simulink model "LQR_SIP_v2"  (R2022b)
settings: Solver=ode4  StartTime=0.0  StopTime=60*5  FixedStep=0.002  RelTol=1e-3  EnableMultiTasking=on
PostLoadFcn:
  | qc_set_target_type(getConfigSet(bdroot, 'QUARC Default Target Configuration'));
undefined symbols (not defined in the file): ALPHA_MAX, ALPHA_MIN, HIL, K, K_EC, K_EP, qc_get_step_size, wcf, XC_MAX, XC_MIN, zetaf
libraries: quarc_library x9, simulink_extras x3
Description:
  | This example is a simple analog loopback test. It sends a signal to analog output
  | channel #0 and then reads analog input channel #0. Wire analog output #0 to analog
  | input #0 to see the signal on the Scope. Change the amplitude of the signal and see
  | the change occur on the Scope.
settings Model: SimulationMode=external  ExtModeTrigDuration=10000  Creator=drmadill  LastModifiedBy=tst2753
settings SolverCC: AlgebraicLoopSolver=TrustRegion  PositivePriorityOrder=on
settings DataIOCC: LimitDataPoints=on  SaveFormat=Array  SignalLoggingSaveFormat=ModelDataLogs  InspectSignalLogs=on  ReturnWorkspaceOutputs=off
settings OptimizationCC: ExpressionDepthLimit=2147483647  InitFltsAndDblsToZero=on
settings DebuggingCC: SaveWithParameterizedLinksMsg=none  UnderspecifiedInitializationDetection=Classic  MergeDetectMultiDrivingBlocksExec=none  SolverPrmCheckMsg=warning  FcnCallInpInsideContextMsg=warning  UnconnectedInputMsg=warning  UnconnectedOutputMsg=warning  UnconnectedLineMsg=warning  StateNameClashWarn=warning  SFUnexpectedBacktrackingDiag=warning  SFNoUnconditionalDefaultTransitionDiag=warning  SFMachineParentedDataDiag=warning  ArithmeticOperatorsInVariantConditions=warning
settings ModelReferenceCC: EnableRefExpFcnMdlSchedulingChecks=on  PropagateSignalLabelsOutOfModel=off
settings SFSimCC: SimUseLocalCustomCode=off  CustomCodeUndefinedFunction=UseInterfaceOnly
settings RTWCC: Description=QUARC Win64 Target Using Toolchain  SystemTargetFile=quarc_win64.tlc  TemplateMakefile=quarc_default_tmf  RTWUseLocalCustomCode=off  Toolchain=QUARC win64 | nmake (64-bit Windows)  BuildConfiguration=Faster Runs
settings CodeAppCC: StateflowObjectComments=on
settings STFCustomTargetCC: ConcurrentExecutionCompliant=on  GRTInterface=on  UseToolchainInfoCompliant=on  SystemTargetFile=quarc_win64.tlc
settings GRTTargetCC: TargetLangStandard=C89/C90 (ANSI)  ParMdlRefBuildCompliant=off  CompOptLevelCompliant=off  CombineOutputUpdateFcns=off  MatFileLogging=off  CPPClassGenCompliant=off  GRTInterface=on  ExtMode=on  ExtModeMexFile=quarc_comm
settings ConfigComp: CovMetricSettings=dw  CovSaveCumulativeToWorkspaceVar=on  CovSaveSingleToWorkspaceVar=on  CovExternalEMLEnable=off

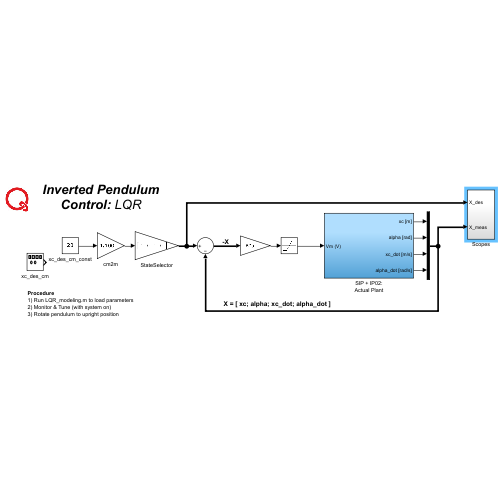
[thumbnail: Simulink's stored preview of the top-level diagram]
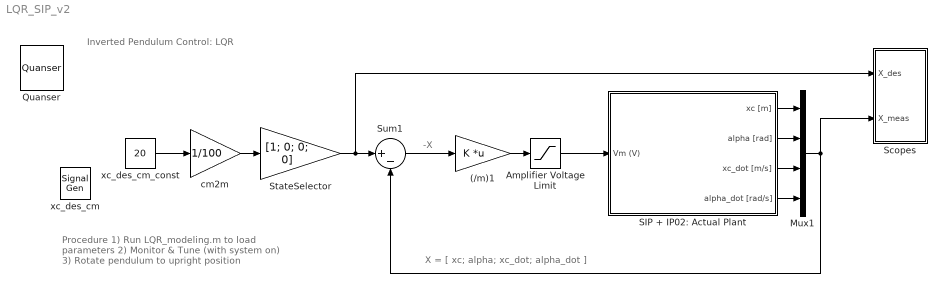
== system LQR_SIP_v2 ==
  note: X = [ xc; alpha; xc_dot; alpha_dot ]
  note: -X
  note: Procedure
      | 1) Run LQR_modeling.m to load parameters
      | 2) Monitor & Tune (with system on)
      | 3) Rotate pendulum to upright position
  note: Inverted Pendulum Control: LQR
  (/m)1 : Gain  Gain=K  Multiplication=Matrix(K*u)  SaturateOnIntegerOverflow=on  OutDataTypeStr=Inherit: Same as input  ParamDataTypeStr=Inherit: Same as input
  Amplifier Voltage Limit : Saturate  UpperLimit=10  LowerLimit=-10
  Mux1 : Mux
  Quanser : quarc_library/Logos/Quanser
  SIP + IP02: Actual Plant : Subsystem
  Scopes : Subsystem
  StateSelector : Gain  Gain=[1; 0; 0; 0]  SaturateOnIntegerOverflow=on  OutDataTypeStr=Inherit: Same as input  ParamDataTypeStr=Inherit: Same as input
  Sum1 : Sum  Inputs=|+-  InputSameDT=on  SaturateOnIntegerOverflow=on  OutDataTypeStr=Inherit: Same as first input
  cm2m : Gain  Gain=1/100  SaturateOnIntegerOverflow=on  OutDataTypeStr=Inherit: Same as input  ParamDataTypeStr=Inherit: Same as input
  xc_des_cm : SignalGenerator  Amplitude=20  Frequency=0.15
  xc_des_cm_const : Constant  Value=20
  wires:
  (/m)1/1 -> Amplifier Voltage Limit/1
  SIP + IP02: Actual Plant/3(xc_dot [m/s]) -> Mux1/3
  cm2m/1 -> StateSelector/1
  StateSelector/1 -> Sum1/1, Scopes/1(X_des)
  Amplifier Voltage Limit/1 -> SIP + IP02: Actual Plant/1(Vm (V))
  Sum1/1 -> (/m)1/1
  SIP + IP02: Actual Plant/4(alpha_dot [rad/s]) -> Mux1/4
  Mux1/1 -> Scopes/2(X_meas), Sum1/2
  SIP + IP02: Actual Plant/1(xc [m]) -> Mux1/1
  SIP + IP02: Actual Plant/2(alpha [rad]) -> Mux1/2
  xc_des_cm_const/1 -> cm2m/1

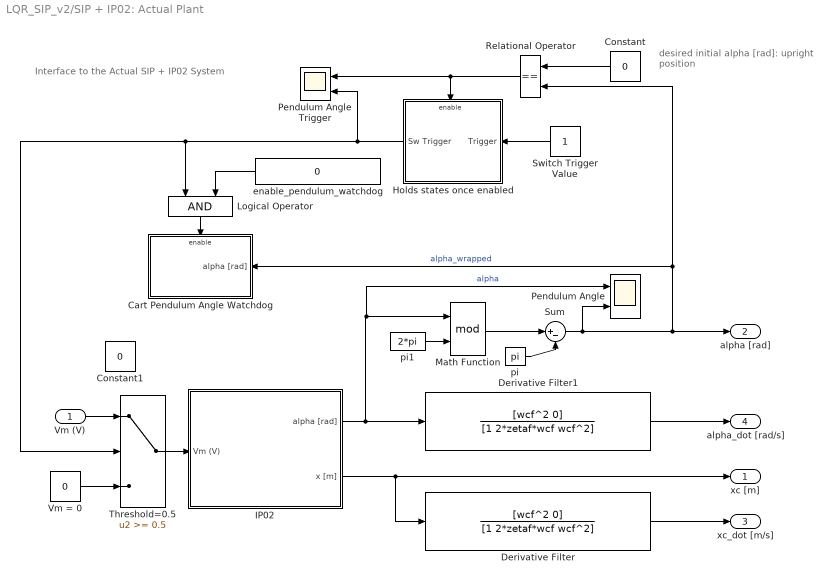
== system LQR_SIP_v2/SIP + IP02: Actual Plant ==
  note: Interface to the Actual
      | SIP + IP02 System
  note: desired initial alpha [rad]:
      | upright position
  Vm (V) : Inport
  Cart Pendulum Angle Watchdog : Subsystem  TreatAsAtomicUnit=on
  Constant : Constant  Value=0
  Constant1 : Constant  Value=0
  Derivative Filter : TransferFcn  Numerator=[wcf^2 0]  Denominator=[1 2*zetaf*wcf wcf^2]
  Derivative Filter1 : TransferFcn  Numerator=[wcf^2 0]  Denominator=[1 2*zetaf*wcf wcf^2]
  Holds states once enabled : Subsystem  TreatAsAtomicUnit=on
  "IP02 " : Subsystem
  Logical Operator : Logic
  Math Function : Math  Operator=mod  SignedPower=on
  Pendulum Angle : Scope  NumInputPorts=2
  Pendulum Angle Trigger : Scope  NumInputPorts=2
  Relational Operator : RelationalOperator  Operator===  OutDataTypeStr=boolean
  Sum : Sum  Inputs=|+-  InputSameDT=on  SaturateOnIntegerOverflow=on  OutDataTypeStr=Inherit: Same as first input
  Switch Trigger Value : Constant  OutDataTypeStr=boolean
  Threshold=0.5 : Switch  Threshold=0.5
  Vm = 0 : Constant  Value=0
  enable_pendulum_watchdog : Constant  Value=0  OutDataTypeStr=boolean
  pi : Constant  Value=pi
  pi1 : Constant  Value=2*pi
  xc [m] : Outport  InitialOutput=0
  alpha [rad] : Outport  Port=2  InitialOutput=0
  xc_dot [m/s] : Outport  Port=3  InitialOutput=0
  alpha_dot [rad/s] : Outport  Port=4  InitialOutput=0
  wires:
  "IP02 "/2(x [m]) -> Derivative Filter/1, xc [m]/1
  Derivative Filter1/1 -> alpha_dot [rad/s]/1
  "IP02 "/1(alpha [rad]) -> Pendulum Angle/1, Math Function/1, Derivative Filter1/1  "alpha"
  Derivative Filter/1 -> xc_dot [m/s]/1
  pi1/1 -> Math Function/2
  Constant/1 -> Relational Operator/1
  Switch Trigger Value/1 -> Holds states once enabled/1(Trigger)
  Relational Operator/1 -> Pendulum Angle Trigger/1, Holds states once enabled/Enable
  Holds states once enabled/1(Sw Trigger) -> Pendulum Angle Trigger/2, Threshold=0.5/2, Logical Operator/1
  Vm = 0/1 -> Threshold=0.5/3
  pi/1 -> Sum/2
  Sum/1 -> Pendulum Angle/2, alpha [rad]/1, Relational Operator/2, Cart Pendulum Angle Watchdog/1(alpha [rad])  "alpha_wrapped"
  Math Function/1 -> Sum/1
  Logical Operator/1 -> Cart Pendulum Angle Watchdog/Enable
  enable_pendulum_watchdog/1 -> Logical Operator/2
  Vm (V)/1 -> Threshold=0.5/1
  Threshold=0.5/1 -> "IP02 "/1(Vm (V))

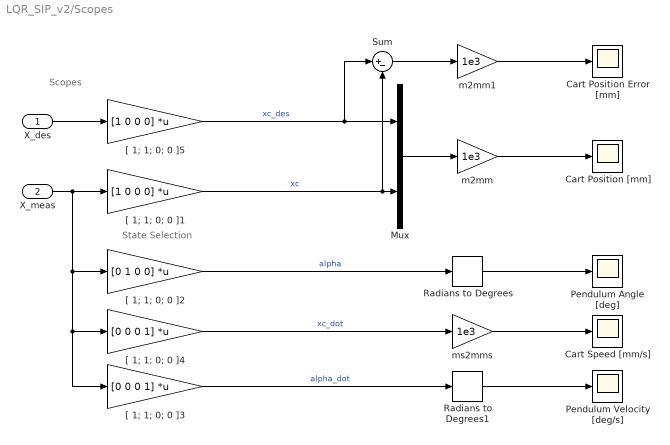
== system LQR_SIP_v2/Scopes ==
  note: State Selection
  note: Scopes
  X_des : Inport
  X_meas : Inport  Port=2
  Cart Position Error [mm] : Scope
  Cart Position [mm] : Scope
  Cart Speed [mm/s] : Scope
  Mux : Mux  Inputs=2
  Pendulum Angle [deg] : Scope
  Pendulum Velocity [deg/s] : Scope
  Radians to Degrees : simulink_extras/Transformations/Radians to Degrees
  Radians to Degrees1 : simulink_extras/Transformations/Radians to Degrees
  Sum : Sum  Inputs=|+-
  "[ 1; 1; 0; 0 ]1" : Gain  Gain=[1 0 0 0]  Multiplication=Matrix(K*u)  SaturateOnIntegerOverflow=on  OutDataTypeStr=Inherit: Same as input  ParamDataTypeStr=Inherit: Same as input
  "[ 1; 1; 0; 0 ]2" : Gain  Gain=[0 1 0 0]  Multiplication=Matrix(K*u)  SaturateOnIntegerOverflow=on  OutDataTypeStr=Inherit: Same as input  ParamDataTypeStr=Inherit: Same as input
  "[ 1; 1; 0; 0 ]3" : Gain  Gain=[0 0 0 1]  Multiplication=Matrix(K*u)  SaturateOnIntegerOverflow=on  OutDataTypeStr=Inherit: Same as input  ParamDataTypeStr=Inherit: Same as input
  "[ 1; 1; 0; 0 ]4" : Gain  Gain=[0 0 0 1]  Multiplication=Matrix(K*u)  SaturateOnIntegerOverflow=on  OutDataTypeStr=Inherit: Same as input  ParamDataTypeStr=Inherit: Same as input
  "[ 1; 1; 0; 0 ]5" : Gain  Gain=[1 0 0 0]  Multiplication=Matrix(K*u)  SaturateOnIntegerOverflow=on  OutDataTypeStr=Inherit: Same as input  ParamDataTypeStr=Inherit: Same as input
  m2mm : Gain  Gain=1e3  SaturateOnIntegerOverflow=on  OutDataTypeStr=Inherit: Same as input  ParamDataTypeStr=Inherit: Same as input
  m2mm1 : Gain  Gain=1e3  SaturateOnIntegerOverflow=on  OutDataTypeStr=Inherit: Same as input  ParamDataTypeStr=Inherit: Same as input
  ms2mms : Gain  Gain=1e3  SaturateOnIntegerOverflow=on  OutDataTypeStr=Inherit: Same as input  ParamDataTypeStr=Inherit: Same as input
  wires:
  Mux/1 -> m2mm/1
  m2mm/1 -> Cart Position [mm]/1
  "[ 1; 1; 0; 0 ]1"/1 -> Sum/2, Mux/2  "xc"
  X_des/1 -> "[ 1; 1; 0; 0 ]5"/1
  X_meas/1 -> "[ 1; 1; 0; 0 ]1"/1, "[ 1; 1; 0; 0 ]3"/1, "[ 1; 1; 0; 0 ]4"/1, "[ 1; 1; 0; 0 ]2"/1
  Radians to Degrees/1 -> Pendulum Angle [deg]/1
  "[ 1; 1; 0; 0 ]5"/1 -> Sum/1, Mux/1  "xc_des"
  "[ 1; 1; 0; 0 ]2"/1 -> Radians to Degrees/1  "alpha"
  m2mm1/1 -> Cart Position Error [mm]/1
  Sum/1 -> m2mm1/1
  "[ 1; 1; 0; 0 ]3"/1 -> Radians to Degrees1/1  "alpha_dot"
  Radians to Degrees1/1 -> Pendulum Velocity [deg/s]/1
  ms2mms/1 -> Cart Speed [mm/s]/1
  "[ 1; 1; 0; 0 ]4"/1 -> ms2mms/1  "xc_dot"

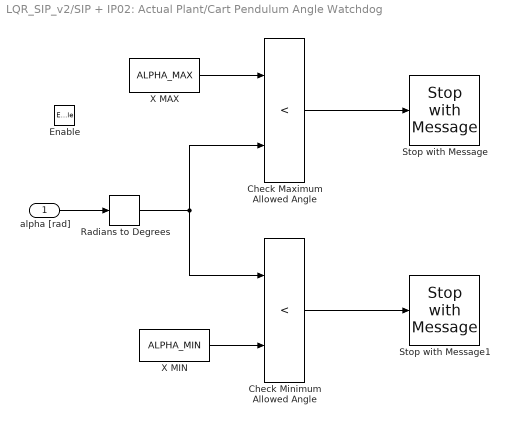
== system LQR_SIP_v2/SIP + IP02: Actual Plant/Cart Pendulum Angle Watchdog ==
  alpha [rad] : Inport
  Enable : EnablePort
  Check Maximum Allowed Angle : RelationalOperator  Operator=<
  Check Minimum Allowed Angle : RelationalOperator  Operator=<
  Radians to Degrees : simulink_extras/Transformations/Radians to Degrees
  Stop with Message : quarc_library/Sinks/Error Handling/Stop with Message  message_type=Fixed error message  message_icon=Error  message=Maximum alpha Reached.
  Stop with Message1 : quarc_library/Sinks/Error Handling/Stop with Message  message_type=Fixed error message  message_icon=Error  message=Minimum alpha Reached.
  X MAX : Constant  Value=ALPHA_MAX
  X MIN : Constant  Value=ALPHA_MIN
  wires:
  X MAX/1 -> Check Maximum Allowed Angle/1
  Check Minimum Allowed Angle/1 -> Stop with Message1/1
  X MIN/1 -> Check Minimum Allowed Angle/2
  alpha [rad]/1 -> Radians to Degrees/1
  Check Maximum Allowed Angle/1 -> Stop with Message/1
  Radians to Degrees/1 -> Check Maximum Allowed Angle/2, Check Minimum Allowed Angle/1

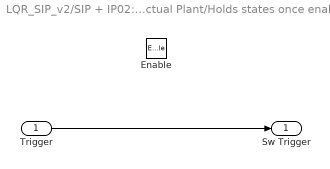
== system LQR_SIP_v2/SIP + IP02: Actual Plant/Holds states once enabled ==
  Trigger : Inport  OutDataTypeStr=boolean
  Enable : EnablePort
  Sw Trigger : Outport  OutDataTypeStr=boolean  InitialOutput=[0]
  wires:
  Trigger/1 -> Sw Trigger/1

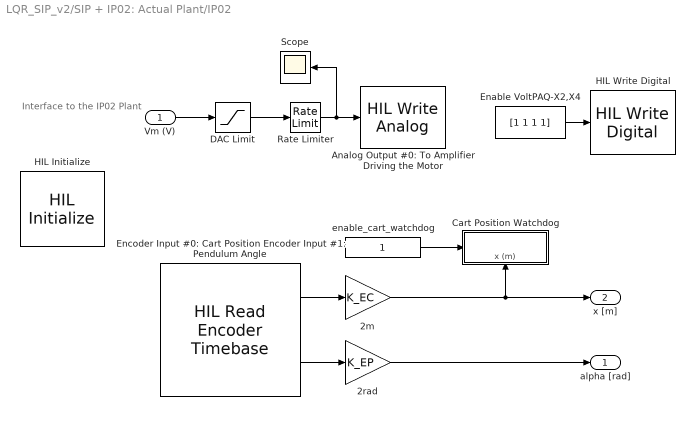
== system LQR_SIP_v2/SIP + IP02: Actual Plant/IP02  ==
  note: Interface to the IP02 Plant
  Vm (V) : Inport
  2m : Gain  Gain=K_EC  SaturateOnIntegerOverflow=on  OutDataTypeStr=Inherit: Same as input  ParamDataTypeStr=Inherit: Same as input
  2rad : Gain  Gain=K_EP  SaturateOnIntegerOverflow=on  OutDataTypeStr=Inherit: Same as input  ParamDataTypeStr=Inherit: Same as input
  Analog Output #0: To Amplifier Driving the Motor : quarc_library/Data Acquisition/Generic/Immediate I//O/HIL Write Analog  Tag=unassigned  object_name=HIL-2  channels=0  sample_time=-1  active=on  vector_input=on
  Cart Position Watchdog : Subsystem  TreatAsAtomicUnit=on
  DAC Limit : Saturate  UpperLimit=10  LowerLimit=-10
  Enable VoltPAQ-X2,X4 : Constant  Value=[1 1 1 1]
  Encoder Input #0: Cart Position Encoder Input #1: Pendulum Angle : quarc_library/Data Acquisition/Generic/Timebases/HIL Read Encoder Timebase  Tag=unassigned  object_name=HIL-2  clock=0  channels=[0 1]  active=on  vector_output=off  data_type_mode=Inherit via back propagation  data_type=double  overflow_mode=Error on overflow  samples_in_buffer=max(ceil(1/qc_get_step_size), 1)
  HIL Initialize : quarc_library/Data Acquisition/Generic/Configuration/HIL Initialize  object_name=HIL-2  board_type=q2_usb  board_number=0  board_options=d0=digital;d1=digital;led=auto;update_rate=normal  exclusive=off  active=off  hardware_clocks=[0:2]  clock_modes=[]  initial_clock_frequencies=[]  set_clock_params_at_start=off  set_clock_params_at_switch_in=off  set_clock_frequencies_at_start=off  set_clock_frequencies_at_switch_in=off  analog_input_channels=[0:1]  analog_input_configurations=[]  analog_input_maximums=10  analog_input_minimums=-10  set_analog_input_params_at_start=on  set_analog_input_params_at_switch_in=off  analog_output_channels=[0:1]  analog_output_maximums=10  analog_output_minimums=-10  initial_analog_outputs=[0]  final_analog_outputs=[0]  watchdog_analog_outputs=0  set_analog_output_params_at_start=on  set_analog_output_params_at_switch_in=off  set_analog_outputs_at_start=on  set_analog_outputs_at_switch_in=off  set_analog_outputs_at_terminate=on  set_analog_outputs_at_switch_out=off  set_analog_outputs_on_watchdog=off  digital_input_channels=[]  digital_output_channels=[0:7]  digital_output_configuration=[]  initial_digital_outputs=[0]  final_digital_outputs=[0]  watchdog_digital_outputs=[0]  set_digital_output_params_at_start=off  set_digital_output_params_at_switch_in=off  set_digital_outputs_at_start=on  set_digital_outputs_at_switch_in=off  set_digital_outputs_at_terminate=on  set_digital_outputs_at_switch_out=off  set_digital_outputs_on_watchdog=off  encoder_channels=[0:1]  quadrature=[4]  encoder_filter_frequency=[]  initial_encoder_counts=[0]  set_encoder_params_at_start=on  set_encoder_params_at_switch_in=off  set_encoder_counts_at_start=on  set_encoder_counts_at_switch_in=off  pwm_channels=[]  pwm_modes=[0]  pwm_frequency=1/0.020  pwm_configuration=[]  pwm_alignment=[]  pwm_polarity=[]  pwm_leading_deadband=[]  pwm_trailing_deadband=[]  initial_pwm_outputs=[0]  final_pwm_outputs=[0]  watchdog_pwm_outputs=[0]  set_pwm_params_at_start=on  set_pwm_params_at_switch_in=off  set_pwm_outputs_at_start=on  set_pwm_outputs_at_switch_in=off  set_pwm_outputs_at_terminate=on  set_pwm_outputs_at_switch_out=off  set_pwm_outputs_on_watchdog=off  other_output_channels=[]  initial_other_outputs=[]  final_other_outputs=[]  watchdog_other_outputs=[]  set_other_outputs_at_start=off  set_other_outputs_at_switch_in=off  set_other_outputs_at_terminate=off  set_other_outputs_at_switch_out=off  set_other_outputs_on_watchdog=off
  HIL Write Digital : quarc_library/Data Acquisition/Generic/Immediate I//O/HIL Write Digital  object_name=HIL-2  channels=[0:3]  sample_time=-1  active=off  vector_input=on
      settings: SourceProductName=QUARC Targets
  Rate Limiter : RateLimiter  RisingSlewLimit=100  FallingSlewLimit=-100  SampleTimeMode=inherited
  Scope : Scope
  enable_cart_watchdog : Constant
  alpha [rad] : Outport  InitialOutput=0
  x [m] : Outport  Port=2  InitialOutput=0
  wires:
  Encoder Input #0: Cart Position Encoder Input #1: Pendulum Angle/1 -> 2m/1
  2m/1 -> Cart Position Watchdog/1(x (m)), x [m]/1
  Vm (V)/1 -> DAC Limit/1
  Encoder Input #0: Cart Position Encoder Input #1: Pendulum Angle/2 -> 2rad/1
  2rad/1 -> alpha [rad]/1
  DAC Limit/1 -> Rate Limiter/1
  Enable VoltPAQ-X2,X4/1 -> HIL Write Digital/1
  Rate Limiter/1 -> Scope/1, Analog Output #0: To Amplifier Driving the Motor/1
  enable_cart_watchdog/1 -> Cart Position Watchdog/Enable

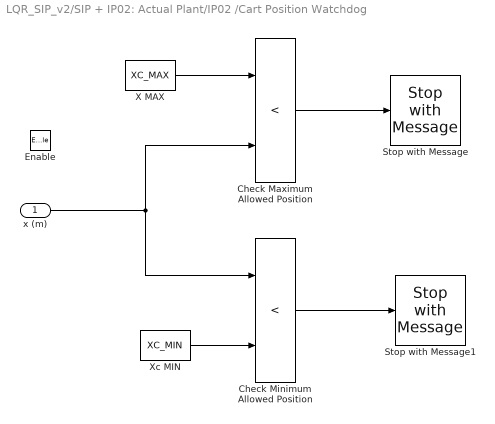
== system LQR_SIP_v2/SIP + IP02: Actual Plant/IP02 /Cart Position Watchdog ==
  x (m) : Inport
  Enable : EnablePort
  Check Maximum Allowed Position : RelationalOperator  Operator=<
  Check Minimum Allowed Position : RelationalOperator  Operator=<
  Stop with Message : quarc_library/Sinks/Error Handling/Stop with Message  message_type=Fixed error message  message_icon=Error  message=Maximum x_c Reached.
  Stop with Message1 : quarc_library/Sinks/Error Handling/Stop with Message  message_type=Fixed error message  message_icon=Error  message=Minimum x_c Reached.
  X MAX : Constant  Value=XC_MAX
  Xc MIN : Constant  Value=XC_MIN
  wires:
  Check Maximum Allowed Position/1 -> Stop with Message/1
  x (m)/1 -> Check Minimum Allowed Position/1, Check Maximum Allowed Position/2
  Xc MIN/1 -> Check Minimum Allowed Position/2
  Check Minimum Allowed Position/1 -> Stop with Message1/1
  X MAX/1 -> Check Maximum Allowed Position/1
